simulink model "gaitPlayBack"  (R2016b)
settings: Solver=FixedStepAuto  StartTime=0.0  StopTime=9  FixedStep=0.001  RelTol=1e-3
values from neighbouring files (symbols this model uses):
  angleHip = [0.188616386175 0.188616044685 0.188615021228 0.188613317334 0.188610934543 0.188607874404 0.188604138478 0.188599728335 0.188594645555 0.188588891728 0.188582468453 0.188575377339 ... (3000 elements, 3000x1)]    [angleHip.mat]
settings Model: Creator=Taeke  LastModifiedBy=Taeke

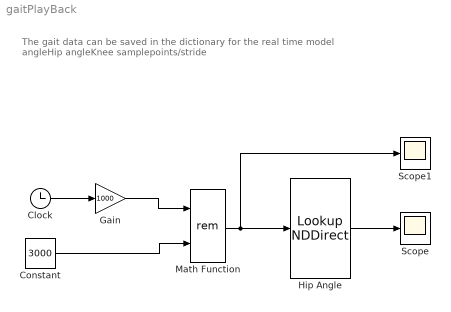
== system gaitPlayBack ==
  note: The gait data can be saved in the dictionary for the real time model
      | angleHip
      | angleKnee
      | samplepoints/stride
  Clock : Clock
      settings: Decimation=1000
  Constant : Constant  Value=3000
  Gain : Gain  Gain=1000
  Hip Angle : LookupNDDirect  NumberOfTableDimensions=1  Table=angleHip
  Math Function : Math  Operator=rem  SaturateOnIntegerOverflow=on
  Scope : Scope
  Scope1 : Scope
  wires:
  Hip Angle/1 -> Scope/1
  Clock/1 -> Gain/1
  Gain/1 -> Math Function/1
  Math Function/1 -> Scope1/1, Hip Angle/1
  Constant/1 -> Math Function/2
